simulink model "kalman_filter_block"  (R2014b)
settings: Solver=ode45  StartTime=0.0  StopTime=10.0  RelTol=1e-3
undefined symbols (not defined in the file): A_kalman_fourbar_gear, B_kalman_fourbar_gear, C_kalman_fourbar_gear, d_vertical_com, Discrete, initial_dx_estimate, k_sea, kalman_load_to_deflect_transmission, LEG_MTR_GEAR_RATIO, max_absolute_measurement_innovation, P0_kalman_fourbar_gear, Q_kalman_rotor_torque, Q_kalman_spring_torque, Q_kalman_trunk_torque, R_kalman_absolute_fail, R_kalman_absolute_normal, R_kalman_incremental_loaded, R_kalman_incremental_unloaded, sample_time, Time
libraries: ctrlSharedLib x4
settings Model: Creator=wmartin  LastModifiedBy=wmartin

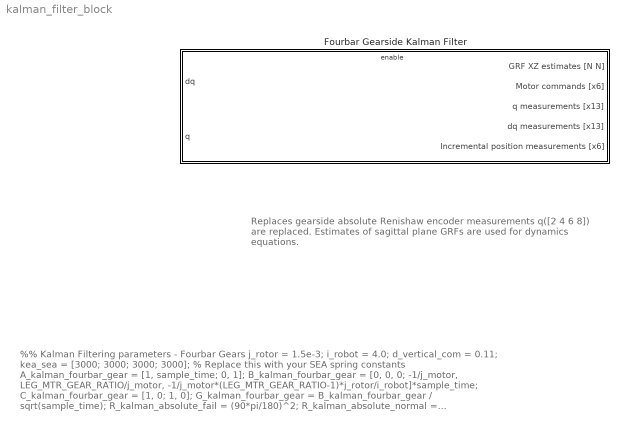
== system kalman_filter_block ==
  note: %% Kalman Filtering parameters - Fourbar Gears
      | j_rotor = 1.5e-3;
      | i_robot = 4.0;
      | d_vertical_com = 0.11;
      | kea_sea = [3000; 3000; 3000; 3000]; % Replace this with your SEA spring constants
      | A_kalman_fourbar_gear = [1, sample_time; 0, 1];
      | B_kalman_fourbar_gear = [0, 0, 0; -1/j_motor, LEG_MTR_GEAR_RATIO/j_motor, -1/j_motor*(LEG_MTR_GEAR_RATIO-1)*j_rotor/i_robot]*sample_time;
      | C_kalman_fourbar_gear = [1, 0; 1, 0];
      | G_kalman_fourbar_gear = B_kalman_fourbar_gear / sqrt(sample_time);
      | R_kalman_absolute_fail = (90*pi/180)^2;
      | R_kalman_absolute_normal = (10^-3*pi/180)^2;
      | R_kalman_incremental_unloaded = (5*10^-3*pi/180)^2 + (LEG_INC_ENCODER_RAD_PER_TICK)^2;
      | R_kalman_incremental_loaded = (2.5*pi/180)^2 + (LEG_INC_ENCODER_RAD_PER_TICK)^2;
      | Q_kalman_spring_torque = 20^2;
      | Q_kalman_rotor_torque = 5^2;
      | Q_kalman_trunk_torque = 0.2^2*Q_kalman_GRF + 4*Q_kalman_rotor_torque + 4*Q_kalman_spring_torque;
      | P0_kalman_fourbar_gear = diag([R_kalman_absolute_normal, 2*R_kalman_absolute_normal/sample_time^2]);
      | max_absolute_measurement_innovation = 15*pi/180;
      | kalman_load_to_deflect_transmission = 500; % Nm
  note: Replaces gearside absolute Renishaw encoder measurements
      |
      | q([2 4 6 8]) are replaced.
      |
      | Estimates of sagittal plane GRFs are used for dynamics equations.
  Fourbar Gearside Kalman Filter : Subsystem

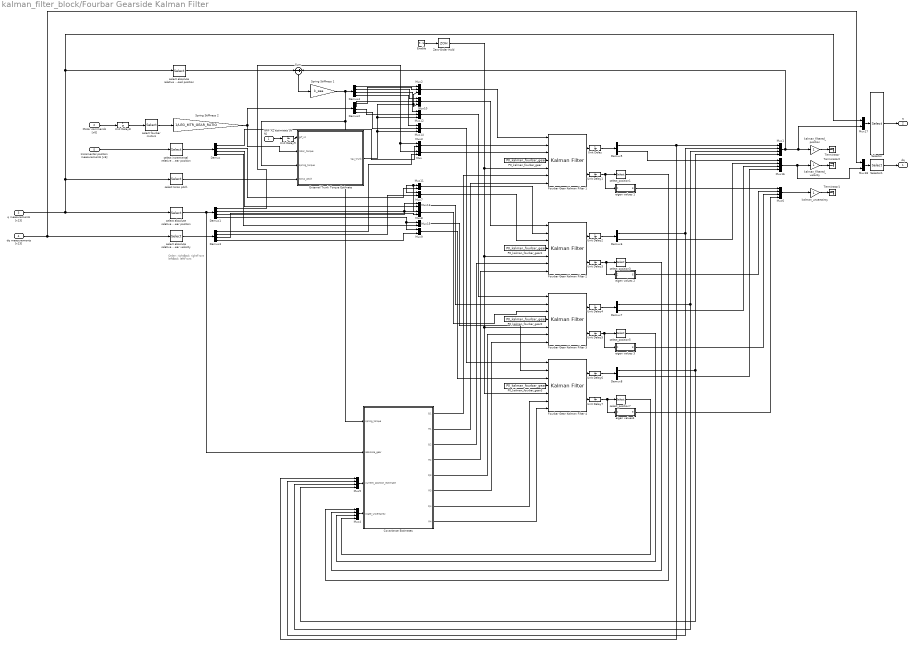
== system kalman_filter_block/Fourbar Gearside Kalman Filter ==
  note: Order:
      | rightBack
      | rightFront
      | leftBack
      | leftFront
  GRF XZ estimates [N N] : Inport  SampleTime=sample_time
  Motor commands [x6] : Inport  Port=2  SampleTime=sample_time
  q measurements [x13] : Inport  Port=3  SampleTime=sample_time
  dq measurements [x13] : Inport  Port=4  SampleTime=sample_time
  Incremental position measurements [x6] : Inport  Port=5  SampleTime=sample_time
  Enable : EnablePort  ShowOutputPort=on
  Covariance Estimates : MATLAB Function  TreatAsAtomicUnit=on
  Demux{,1..4} (5 alike) : Demux
  Demux{5..8} (4 alike) : Demux  Outputs=2
  External Trunk Torque Estimate : MATLAB Function  TreatAsAtomicUnit=on
  Fourbar Gear Kalman Filter {1..4} (4 alike) : ctrlSharedLib/Kalman Filter  TimeDomain=Discrete-Time  UseCurrentEstimator=on  ModelSource=Individual A, B, C, D matrices  ModelSourceVariable=A_kf  A=A_kalman_fourbar_gear  B=B_kalman_fourbar_gear  C=C_kalman_fourbar_gear  D=0  NumberOfStates=2  NumberOfInputs=1  NumberOfOutputs=2  InitialEstimateSource=Input port  X0=initial_dx_estimate  P0=P0_kalman_transverse  UseK=off  UseGH=on  NumberOfProcessNoiseInputs=1  G=G_kalman_fourbar_gear  TimeInvariantG=on  H=0  TimeInvariantH=on  Q=1  TimeInvariantQ=off  R=1  TimeInvariantR=off  N=0  TimeInvariantN=on  AddInputPort=on  AddEnablePort=off  ExternalReset=Either  OutputEstimatedY=off  OutputP=on  Ts=sample_time
  Mux{,3,7..9,11,13,15,17..18} (10 alike) : Mux  Inputs=2
  Mux{1,4..6,16} (5 alike) : Mux
  Mux{2,10,12,14} (4 alike) : Mux  Inputs=3
  P0_kalman_fourbar_gear{,1..3} (4 alike) : Constant  Value=P0_kalman_fourbar_gear
  Selector : Selector  InputPortWidth=17  Indices=[1 14 3 15 5 16 7 17 9 10 11 12 13]
  Selector1 : Selector  InputPortWidth=17  Indices=[1 14 3 15 5 16 7 17 9 10 11 12 13]
  Spring Stiffness 1 : Gain  Gain=k_sea
  Spring Stiffness 2 : Gain  Gain=1/LEG_MTR_GEAR_RATIO
  Sum : Sum  Inputs=-|+
  Terminator : Terminator
  Terminator1 : Terminator
  Terminator2 : Terminator
  Unit Delay{,1..9} (10 alike) : UnitDelay  SampleTime=-1
  Zero-Order Hold : ZeroOrderHold  SampleTime=sample_time
  eigen values 1 : MATLAB Function  TreatAsAtomicUnit=on
  eigen values 2 : MATLAB Function  TreatAsAtomicUnit=on
  eigen values 3 : MATLAB Function  TreatAsAtomicUnit=on
  "eigen values4 " : MATLAB Function  TreatAsAtomicUnit=on
  kalman_filtered_position : Gain
  kalman_filtered_velocity : Gain
  kalman_uncertainty : Gain
  select absolute relative gear position : Selector  InputPortWidth=13  Indices=[2 4 6 8]
  select absolute relative gear velocity : Selector  InputPortWidth=13  Indices=[2 4 6 8]
  select absolute relative load position : Selector  InputPortWidth=13  Indices=[2 4 6 8]
  select fourbar motors : Selector  InputPortWidth=6  Indices=[1 2 3 4]
  select incremental relative gear position : Selector  InputPortWidth=6  Indices=[1 2 3 4]
  select torso pitch : Selector  InputPortWidth=13  Indices=[13]
  select_position{1,3,5,7} (4 alike) : Selector  NumberOfDimensions=2  InputPortWidth=2  IndexOptions=Index vector (dialog),Index vector (dialog)  Indices=[1],[1]  OutputSizes=1,1
  dq : Outport
  q : Outport  Port=2
  wires:
  select incremental relative gear position/1 -> Demux/1
  q measurements [x13]/1 -> select absolute relative gear position/1, Mux17/1, select absolute relative load position/1, select torso pitch/1
  Incremental position measurements [x6]/1 -> select incremental relative gear position/1
  Motor commands [x6]/1 -> Unit Delay8/1
  select fourbar motors/1 -> Spring Stiffness 2/1
  P0_kalman_fourbar_gear/1 -> Fourbar Gear Kalman Filter 1/4
  Mux/1 -> Fourbar Gear Kalman Filter 1/3
  select absolute relative gear velocity/1 -> Demux3/1
  dq measurements [x13]/1 -> Mux18/1, select absolute relative gear velocity/1
  Demux3/1 -> Mux/2
  GRF XZ estimates [N N]/1 -> Unit Delay9/1
  Spring Stiffness 1/1 -> Demux4/1, External Trunk Torque Estimate/3(spring_torque), Covariance Estimates/1(spring_torque)
  Fourbar Gear Kalman Filter 1/1 -> Unit Delay/1
  Demux5/1 -> Mux1/1, Mux5/1
  Mux1/1 -> Sum/2, Mux17/2, kalman_filtered_position/1
  select absolute relative load position/1 -> Sum/1
  Sum/1 -> Spring Stiffness 1/1
  External Trunk Torque Estimate/1(tau_trunk) -> Mux2/3, Mux10/3, Mux12/3, Mux14/3
  Demux4/1 -> Mux2/1
  Demux2/1 -> Mux2/2
  Mux2/1 -> Fourbar Gear Kalman Filter 1/1
  Demux/1 -> Mux3/2
  Demux1/1 -> Mux3/1, Mux/1
  Mux3/1 -> Fourbar Gear Kalman Filter 1/2
  Fourbar Gear Kalman Filter 1/2 -> Unit Delay1/1
  Mux4/1 -> Covariance Estimates/4(state_uncertainty)
  select absolute relative gear position/1 -> Covariance Estimates/2(absolute_gear), Demux1/1
  Mux5/1 -> Covariance Estimates/3(current_position_estimate)
  Covariance Estimates/1(Q1) -> Fourbar Gear Kalman Filter 1/6
  Covariance Estimates/2(R1) -> Fourbar Gear Kalman Filter 1/7
  select torso pitch/1 -> External Trunk Torque Estimate/4(torso_pitch)
  select_position1/1 -> Mux4/1
  P0_kalman_fourbar_gear1/1 -> Fourbar Gear Kalman Filter 2/4
  Fourbar Gear Kalman Filter 2/1 -> Unit Delay2/1
  Fourbar Gear Kalman Filter 2/2 -> Unit Delay3/1
  P0_kalman_fourbar_gear2/1 -> Fourbar Gear Kalman Filter 3/4
  Fourbar Gear Kalman Filter 3/1 -> Unit Delay4/1
  Fourbar Gear Kalman Filter 3/2 -> Unit Delay5/1
  P0_kalman_fourbar_gear3/1 -> Fourbar Gear Kalman Filter 4/4
  Fourbar Gear Kalman Filter 4/1 -> Unit Delay6/1
  Fourbar Gear Kalman Filter 4/2 -> Unit Delay7/1
  Covariance Estimates/3(Q2) -> Fourbar Gear Kalman Filter 2/6
  Covariance Estimates/5(Q3) -> Fourbar Gear Kalman Filter 3/6
  Covariance Estimates/7(Q4) -> Fourbar Gear Kalman Filter 4/6
  Covariance Estimates/4(R2) -> Fourbar Gear Kalman Filter 2/7
  Covariance Estimates/6(R3) -> Fourbar Gear Kalman Filter 3/7
  Covariance Estimates/8(R4) -> Fourbar Gear Kalman Filter 4/7
  select_position3/1 -> Mux4/2
  select_position5/1 -> Mux4/3
  select_position7/1 -> Mux4/4
  Demux6/1 -> Mux5/2, Mux1/2
  Demux7/1 -> Mux1/3, Mux5/3
  Demux8/1 -> Mux1/4, Mux5/4
  kalman_filtered_position/1 -> Terminator/1
  Enable/1 -> Zero-Order Hold/1
  Mux7/1 -> Fourbar Gear Kalman Filter 2/3
  Mux8/1 -> Fourbar Gear Kalman Filter 3/3
  Mux9/1 -> Fourbar Gear Kalman Filter 4/3
  Mux10/1 -> Fourbar Gear Kalman Filter 2/1
  Mux11/1 -> Fourbar Gear Kalman Filter 2/2
  Mux13/1 -> Fourbar Gear Kalman Filter 3/2
  Mux12/1 -> Fourbar Gear Kalman Filter 3/1
  Mux15/1 -> Fourbar Gear Kalman Filter 4/2
  Mux14/1 -> Fourbar Gear Kalman Filter 4/1
  Demux3/2 -> Mux7/2
  Demux3/3 -> Mux8/2
  Demux3/4 -> Mux9/2
  Demux1/2 -> Mux7/1, Mux11/1
  Demux1/3 -> Mux13/1, Mux8/1
  Demux1/4 -> Mux9/1, Mux15/1
  Demux/2 -> Mux11/2
  Demux/3 -> Mux13/2
  Demux/4 -> Mux15/2
  Demux4/2 -> Mux10/1
  Demux4/3 -> Mux12/1
  Demux4/4 -> Mux14/1
  Demux2/2 -> Mux10/2
  Demux2/3 -> Mux12/2
  Demux2/4 -> Mux14/2
  kalman_uncertainty/1 -> Terminator1/1
  Mux6/1 -> kalman_uncertainty/1
  kalman_filtered_velocity/1 -> Terminator2/1
  Mux16/1 -> Mux18/2, kalman_filtered_velocity/1
  Demux5/2 -> Mux16/1
  Demux6/2 -> Mux16/2
  Demux7/2 -> Mux16/3
  Demux8/2 -> Mux16/4
  Zero-Order Hold/1 -> Fourbar Gear Kalman Filter 4/5, Fourbar Gear Kalman Filter 3/5, Fourbar Gear Kalman Filter 2/5, Fourbar Gear Kalman Filter 1/5
  Unit Delay1/1 -> eigen values 1/1(Z), select_position1/1
  Unit Delay3/1 -> eigen values 2/1(Z), select_position3/1
  Unit Delay4/1 -> Demux7/1
  Unit Delay7/1 -> "eigen values4 "/1(Z), select_position7/1
  Unit Delay6/1 -> Demux8/1
  Spring Stiffness 2/1 -> Demux2/1, External Trunk Torque Estimate/2(rotor_torque)
  Unit Delay5/1 -> eigen values 3/1(Z), select_position5/1
  eigen values 1/1(E) -> Mux6/1
  eigen values 2/1(E) -> Mux6/2
  eigen values 3/1(E) -> Mux6/3
  "eigen values4 "/1(E) -> Mux6/4
  Unit Delay/1 -> Demux5/1
  Unit Delay2/1 -> Demux6/1
  Mux17/1 -> Selector/1
  Selector/1 -> q/1
  Selector1/1 -> dq/1
  Mux18/1 -> Selector1/1
  Unit Delay8/1 -> select fourbar motors/1
  Unit Delay9/1 -> External Trunk Torque Estimate/1(grf_xz)

== matlab function kalman_filter_block/Fourbar Gearside Kalman Filter/External Trunk Torque Estimate ==
  data: grf_xz input; rotor_torque input; spring_torque input; tau_trunk output; torso_pitch input; d_vertical_com parameter; LEG_MTR_GEAR_RATIO parameter
function tau_trunk = tau_trunk(grf_xz, rotor_torque, spring_torque, torso_pitch, d_vertical_com, LEG_MTR_GEAR_RATIO )
    d = d_vertical_com;
    theta = torso_pitch;
    N = LEG_MTR_GEAR_RATIO;
    tau_trunk = sum(-rotor_torque + -(N-1)/N*spring_torque) + (-d*cos(theta)*grf_xz(1) + d*sin(theta)*grf_xz(2));
end

== matlab function kalman_filter_block/Fourbar Gearside Kalman Filter/Covariance Estimates ==
  data: spring_torque input; absolute_gear input; current_position_estimate input; state_uncertainty input; Q1 output; R1 output; Q2 output; R2 output; R_kalman_absolute_normal parameter; R_kalman_absolute_fail parameter; R_kalman_incremental_unloaded parameter; R_kalman_incremental_loaded parameter; kalman_load_to_deflect_transmission parameter; Q3 output; R3 output; Q4 output; R4 output; max_absolute_measurement_innovation parameter; k_sea parameter; Q_kalman_spring_torque parameter; Q_kalman_rotor_torque parameter; Q_kalman_trunk_torque parameter; sample_time parameter
function [Q1, R1, Q2, R2, Q3, R3, Q4, R4] = covariance( spring_torque, absolute_gear, current_position_estimate, state_uncertainty, R_kalman_absolute_normal, R_kalman_absolute_fail, R_kalman_incremental_unloaded, R_kalman_incremental_loaded, kalman_load_to_deflect_transmission, max_absolute_measurement_innovation, k_sea, Q_kalman_spring_torque, Q_kalman_rotor_torque, Q_kalman_trunk_torque, sample_time)

    persistent previous_absolute_gear
    if isempty(previous_absolute_gear)
        previous_absolute_gear = absolute_gear;
    end
    
    % Measurement covariance
    R_absolute = ones(4,1)*R_kalman_absolute_normal;
    dropped_out = previous_absolute_gear == absolute_gear;
    out_of_range = abs(current_position_estimate - absolute_gear) > max_absolute_measurement_innovation;
    R_absolute(dropped_out | out_of_range) = R_kalman_absolute_fail;
    
    R_incremental_scale = min(abs(spring_torque)/kalman_load_to_deflect_transmission, 1);
    R_incremental = R_incremental_scale*R_kalman_incremental_loaded + (1-R_incremental_scale)*R_kalman_incremental_unloaded;
    
    R1 = diag([R_absolute(1), R_incremental(1)])/sample_time;
    R2 = diag([R_absolute(2), R_incremental(2)])/sample_time;
    R3 = diag([R_absolute(3), R_incremental(3)])/sample_time;
    R4 = diag([R_absolute(4), R_incremental(4)])/sample_time;
    
    % Process noise covariance
    Q_spring_torque = k_sea'.^2.*(state_uncertainty + R_kalman_absolute_normal) + Q_kalman_spring_torque;

    Q1 = diag([Q_spring_torque(1), Q_kalman_rotor_torque, Q_kalman_trunk_torque]);
    Q2 = diag([Q_spring_torque(2), Q_kalman_rotor_torque, Q_kalman_trunk_torque]);
    Q3 = diag([Q_spring_torque(3), Q_kalman_rotor_torque, Q_kalman_trunk_torque]);
    Q4 = diag([Q_spring_torque(4), Q_kalman_rotor_torque, Q_kalman_trunk_torque]);

    previous_absolute_gear = absolute_gear;
end

== matlab function kalman_filter_block/Fourbar Gearside Kalman Filter/eigen values 1 ==
  data: Z input; E output
function E = eigen(Z)
    E = real(eig(Z));
    E = sort(E);
end

== matlab function kalman_filter_block/Fourbar Gearside Kalman Filter/eigen values 2 ==
  data: Z input; E output
function E = eigen(Z)
    E = real(eig(Z));
    E = sort(E);
end

== matlab function kalman_filter_block/Fourbar Gearside Kalman Filter/eigen values 3 ==
  data: Z input; E output
function E = eigen(Z)
    E = real(eig(Z));
    E = sort(E);
end

== matlab function kalman_filter_block/Fourbar Gearside Kalman Filter/eigen values4  ==
  data: Z input; E output
function E = eigen(Z)
    E = real(eig(Z));
    E = sort(E);
end
